simulink model "prepFixedPointController_2020b"  (R2020b)
settings: Solver=VariableStepAuto  StartTime=0.0  StopTime=10.0  RelTol=1e-3
undefined symbols (not defined in the file): data
libraries: mci_models x2
settings Model: Creator=fluky  LastModifiedBy=ematric
settings DebuggingCC: UnconnectedInputMsg=none  UnconnectedOutputMsg=none  UnconnectedLineMsg=none
settings ModelReferenceCC: EnableRefExpFcnMdlSchedulingChecks=off

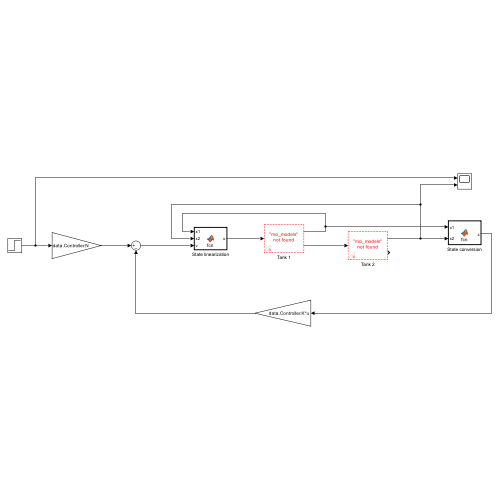
[thumbnail: Simulink's stored preview of the top-level diagram]
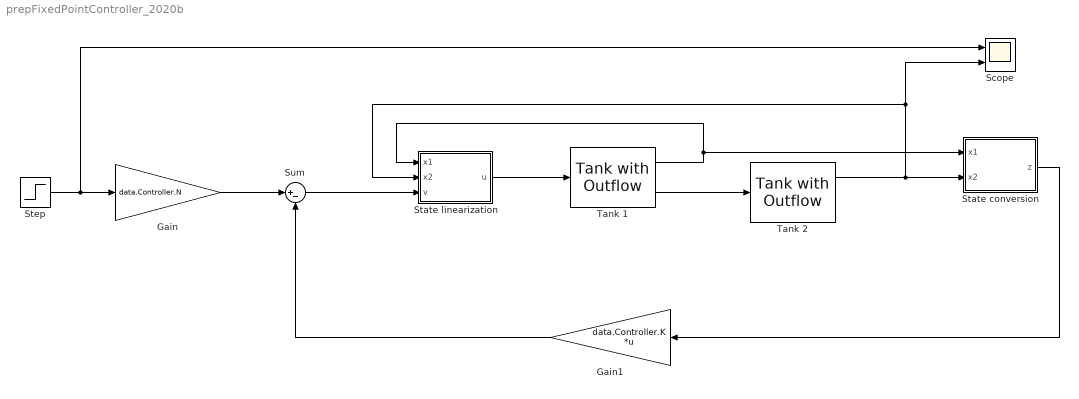
== system prepFixedPointController_2020b ==
  Gain : Gain  Gain=data.Controller.N
  Gain1 : Gain  Gain=data.Controller.K  Multiplication=Matrix(K*u)
  Scope : Scope  NumInputPorts=2
  State conversion : MATLAB Function  TreatAsAtomicUnit=on
  State linearization : MATLAB Function  TreatAsAtomicUnit=on
  Step : Step  Time=10  Before=0.0  After=0.1  SampleTime=0
  Sum : Sum  Inputs=|+-
  Tank 1 : mci_models/Fluid Systems/Tank with Outflow  At=data.At  Ao=data.Aout  rho=data.roh  zeta=data.zeta  g=data.g  h0=data.initHeight
  Tank 2 : mci_models/Fluid Systems/Tank with Outflow  At=data.At  Ao=data.Aout  rho=data.roh  zeta=data.zeta  g=data.g  h0=data.initHeight
  wires:
  Step/1 -> Scope/1, Gain/1
  Gain/1 -> Sum/1
  Sum/1 -> State linearization/3(v)
  State linearization/1(u) -> Tank 1/1
  Tank 1/2 -> Tank 2/1
  Tank 2/1 -> Scope/2, State linearization/2(x2), State conversion/2(x2)
  State conversion/1(z) -> Gain1/1
  Gain1/1 -> Sum/2
  Tank 1/1 -> State linearization/1(x1), State conversion/1(x1)

== matlab function prepFixedPointController_2020b/State conversion ==
  data: x1 input; z output; x2 input; data parameter
function z = fcn(x1, x2, data)
z = [0;0];
z(1) = x2; % is equal to y
z(2) = data.a*sqrt(x1) - data.a*sqrt(x2); % is equal to y_dot

== matlab function prepFixedPointController_2020b/State linearization ==
  data: x1 input; u output; x2 input; v input; data parameter
function u = fcn(x1, x2, v, data)
u = data.roh * data.At * sqrt(x1) * (2*v/data.a + data.a*sqrt(x1/x2));
